simulink model "ThermoDynamicsFMU"  (R2023b)
settings: Solver=FixedStepAuto  StartTime=0.0  StopTime=200  FixedStep=1  RelTol=1e-3
values from neighbouring files (symbols this model uses):
  A = 0.1817    [init_4_sim.m]    (also in startingThermodynamics.m)
  Cp = 1.2552    [init_4_sim.m]    (also in startingThermodynamics.m)
  delta_H = -91200    [init_4_sim.m]    (also in startingThermodynamics.m)
  h = 200.89    [init_4_sim.m]    (also in startingThermodynamics.m)
  rho = 1    [init_4_sim.m]    (also in startingThermodynamics.m)
  T_k0 = 293.15    [init_4_sim.m]
  t_step = 1    [init_4_sim.m]    (also in init_sim2.m; init_sim_suggarferm.m; startingThermodynamics.m)
  Vol = volume    (= 25)    [init_4_sim.m]    (also in startingThermodynamics.m)
settings Model: Creator=20181234  LastModifiedBy=20181234

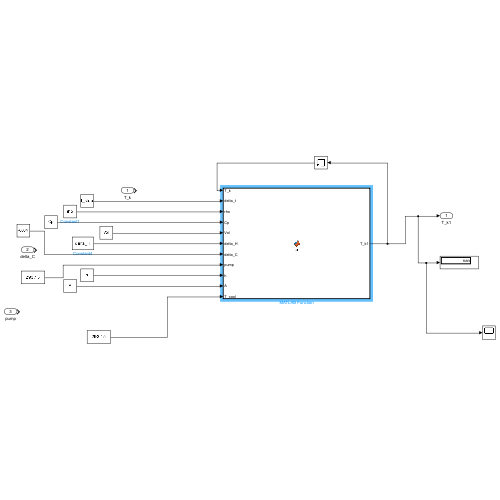
[thumbnail: Simulink's stored preview of the top-level diagram]
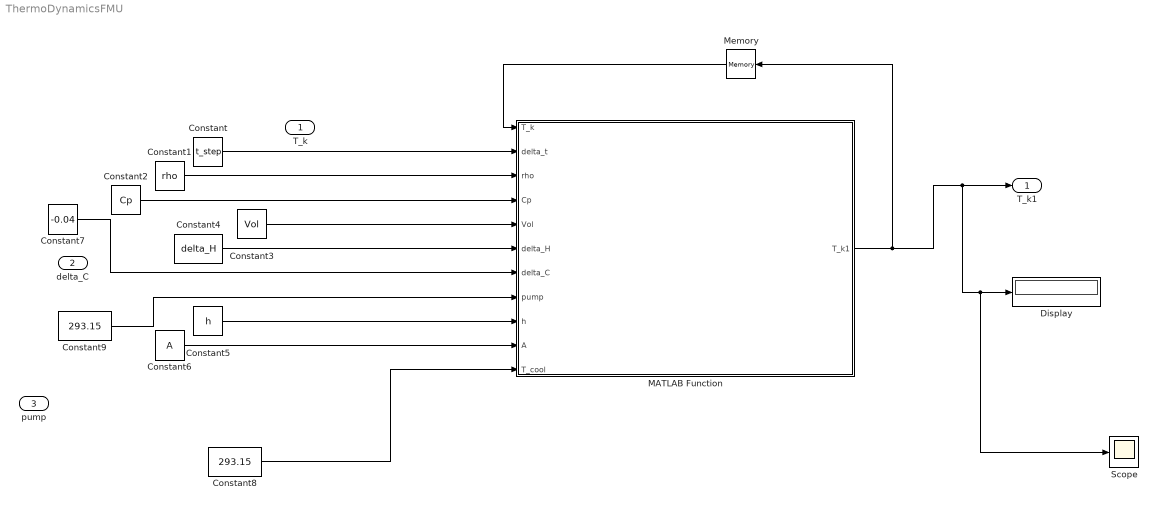
== system ThermoDynamicsFMU ==
  T_k : Inport
  delta_C : Inport  Port=2
  pump : Inport  Port=3
  Constant : Constant  Value=t_step
  Constant1 : Constant  Value=rho
  Constant2 : Constant  Value=Cp
  Constant3 : Constant  Value=Vol
  Constant4 : Constant  Value=delta_H
  Constant5 : Constant  Value=h
  Constant6 : Constant  Value=A
  Constant7 : Constant  Value=-0.04
  Constant8 : Constant  Value=293.15
  Constant9 : Constant  Value=293.15
  Display : Display
  MATLAB Function : MATLAB Function  TreatAsAtomicUnit=on
  Memory : Memory  InitialCondition=T_k0
  Scope : Scope
  T_k1 : Outport
  wires:
  Constant/1 -> MATLAB Function/2(delta_t)
  Constant1/1 -> MATLAB Function/3(rho)
  Constant6/1 -> MATLAB Function/10(A)
  Constant5/1 -> MATLAB Function/9(h)
  Constant4/1 -> MATLAB Function/6(delta_H)
  Constant3/1 -> MATLAB Function/5(Vol)
  Constant2/1 -> MATLAB Function/4(Cp)
  MATLAB Function/1(T_k1) -> Memory/1, Scope/1, Display/1, T_k1/1
  Constant7/1 -> MATLAB Function/7(delta_C)
  Constant9/1 -> MATLAB Function/8(pump)
  Memory/1 -> MATLAB Function/1(T_k)
  Constant8/1 -> MATLAB Function/11(T_cool)

== matlab function ThermoDynamicsFMU/MATLAB Function ==
  data: T_k input; T_k1 output; delta_t input; rho input; Cp input; Vol input; delta_H input; delta_C input; pump input; h input; A input; T_cool input
function T_k1 = fcn(T_k,delta_t, rho, Cp, Vol, delta_H, delta_C, pump, h, A, T_cool)


factor = delta_t / (rho * Cp * Vol);
T_k1 = factor * (-delta_H * delta_C - pump * h * A * (T_k - T_cool)) + T_k;
